simulink model "Arduino_heat_exchanger_PID"  (R2017b)
settings: Solver=VariableStepAuto  StartTime=0.0  StopTime=2400  RelTol=1e-3
values from neighbouring files (symbols this model uses):
  Area = n*A_heat_plate    (= 9.8716)    [heat_exchanger_config.m]    (also in linearization.m = 20)
  cp_H2O = 4190    [heat_exchanger_config.m]    (also in linearization.m)
  cp_wort = 4062    [heat_exchanger_config.m]    (also in linearization.m = 4000)
  HE_delay = 25    [heat_exchanger_config.m]    (also in linearization.m = 5)
  m_H2O = m_wort    (= 10)    [heat_exchanger_config.m]    (also in linearization.m = 1)
  m_wort = 10    [heat_exchanger_config.m]    (also in linearization.m = 1)
  rho_wort = 1.06    [heat_exchanger_config.m]    (also in linearization.m)
  T_H2O_in = 5    [heat_exchanger_config.m]    (also in linearization.m = 10)
  T_wort_in = 95    [heat_exchanger_config.m]    (also in linearization.m = 70)
  U = (m_dot_h_data*cp_wort*(T_wort_in-T_wort_out)*log(Delta_T2/Delta_T1))/     (Area*(Delta_T2-Delta_T1))    [heat_exchanger_config.m]    (also in linearization.m = 1000)
libraries: instrumentlib x3, simulink x1
settings Model: Creator=Alexander  LastModifiedBy=Oscar

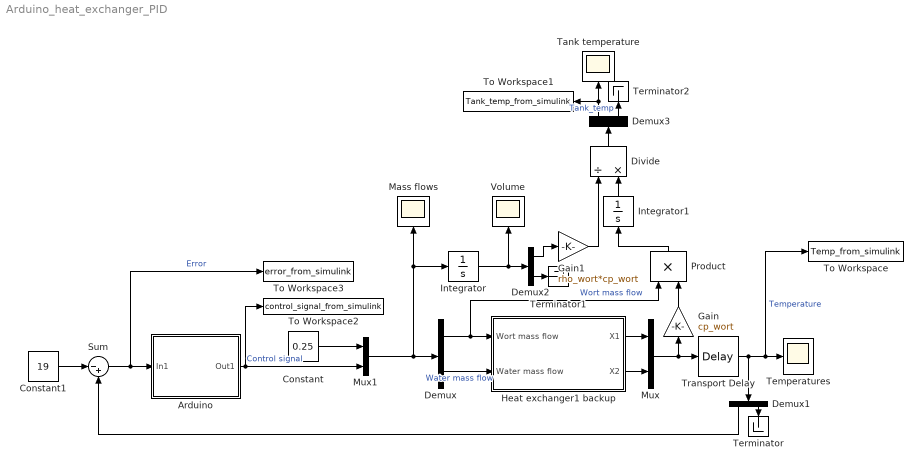
== system Arduino_heat_exchanger_PID ==
  "Arduino " : Subsystem
  Constant : Constant  Value=0.25
  Constant1 : Constant  Value=19
  Demux{,1..3} (4 alike) : Demux  Outputs=2
  Divide : Product  Inputs=/*
  Gain : Gain  Gain=cp_wort
  Gain1 : Gain  Gain=rho_wort*cp_wort
  Heat exchanger1 backup : Subsystem
  Integrator : Integrator
  Integrator1 : Integrator
  Mass flows : Scope
  Mux : Mux  Inputs=2
  Mux1 : Mux  Inputs=2
  Product : Product
  Sum : Sum  Inputs=|-+
  Tank temperature : Scope
  Temperatures : Scope
  Terminator : Terminator
  Terminator1 : Terminator
  Terminator2 : Terminator
  To Workspace : ToWorkspace  VariableName=Temp_from_simulink  SaveFormat=Timeseries  SampleTime=-1
  To Workspace1 : ToWorkspace  VariableName=Tank_temp_from_simulink  SaveFormat=Timeseries  SampleTime=-1
  To Workspace2 : ToWorkspace  VariableName=control_signal_from_simulink  SaveFormat=Timeseries  SampleTime=-1
  To Workspace3 : ToWorkspace  VariableName=error_from_simulink  SaveFormat=Timeseries  SampleTime=-1
  Transport Delay : TransportDelay  DelayTime=HE_delay
  Volume : Scope
  wires:
  Demux/2 -> Heat exchanger1 backup/2(Water mass flow)  "Water mass flow"
  Demux/1 -> Product/1, Heat exchanger1 backup/1(Wort mass flow)  "Wort mass flow"
  Mux/1 -> Gain/1, Transport Delay/1
  Integrator/1 -> Demux2/1, Volume/1
  Transport Delay/1 -> Demux1/1, To Workspace/1, Temperatures/1  "Temperature"
  Demux1/2 -> Terminator/1
  Mux1/1 -> Integrator/1, Mass flows/1, Demux/1
  Constant/1 -> Mux1/1
  Demux1/1 -> Sum/2
  Constant1/1 -> Sum/1
  Heat exchanger1 backup/1(X1) -> Mux/1
  Heat exchanger1 backup/2(X2) -> Mux/2
  Integrator1/1 -> Divide/2
  Gain1/1 -> Divide/1
  Product/1 -> Integrator1/1
  Gain/1 -> Product/2
  Demux2/1 -> Gain1/1
  Demux2/2 -> Terminator1/1
  Demux3/2 -> Terminator2/1
  Divide/1 -> Demux3/1
  Demux3/1 -> Tank temperature/1, To Workspace1/1  "Tank_temp"
  Sum/1 -> To Workspace3/1, "Arduino "/1(In1)  "Error"
  "Arduino "/1(Out1) -> Mux1/2, To Workspace2/1  "Control signal"

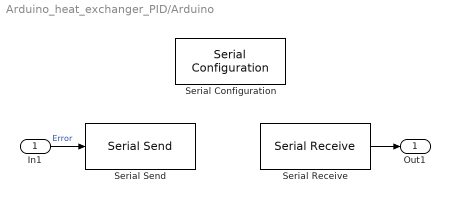
== system Arduino_heat_exchanger_PID/Arduino  ==
  In1 : Inport
  Serial Configuration : instrumentlib/Serial Configuration  Priority=-200000  ComPortMenu=<Please select a port...>  ComPort=<Please select a port...>  BaudRate=9600  DataBits=8  Parity=none  StopBits=1  FlowControl=none  Timeout=10  ByteOrder=LittleEndian
  Serial Receive : instrumentlib/Serial Receive  ComPortMenu=<Please select a port...>  ComPort=<Please select a port...>  Terminator=<none>  DataSize=[1 1]  DataType=uint8  EnableBlockingMode=on  ActionDataUnavailable=Output last received value  CustomValue=0  SampleTime=0.01
  Serial Send : instrumentlib/Serial Send  ComPortMenu=<Please select a port...>  ComPort=<Please select a port...>  Terminator=<none>  EnableBlockingMode=on
  Out1 : Outport
  wires:
  In1/1 -> Serial Send/1  "Error"
  Serial Receive/1 -> Out1/1

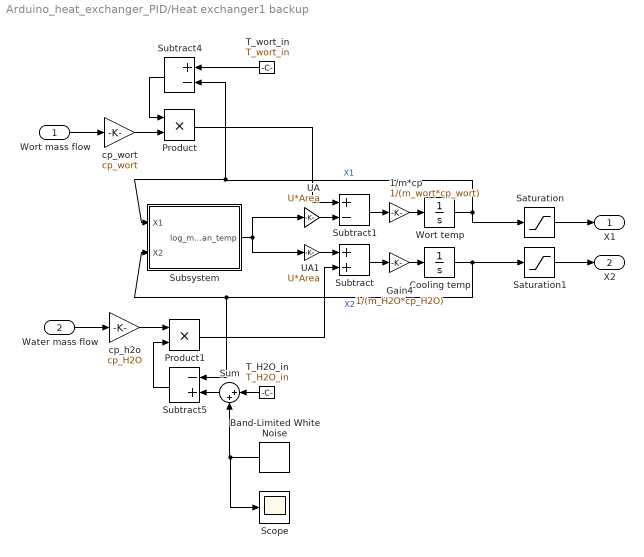
== system Arduino_heat_exchanger_PID/Heat exchanger1 backup ==
  Wort mass flow : Inport
  Water mass flow : Inport  Port=2
  "1/m*cp " : Gain  Gain=1/(m_wort*cp_wort)
  Band-Limited White Noise : simulink/Sources/Band-Limited White Noise  Cov=[5]  Ts=100  seed=[23341]
  Cooling temp : Integrator  InitialCondition=T_H2O_in-0.1
  Gain4 : Gain  Gain=1/(m_H2O*cp_H2O)
  Product : Product
  Product1 : Product
  Saturation : Saturate  UpperLimit=T_wort_in  LowerLimit=T_H2O_in
  Saturation1 : Saturate  UpperLimit=T_wort_in  LowerLimit=T_H2O_in
  Scope : Scope
  Subsystem : Subsystem
  Subtract : Sum
  Subtract1 : Sum  Inputs=+-
  Subtract4 : Sum  Inputs=+-
  Subtract5 : Sum  Inputs=-+
  Sum : Sum  Inputs=|++
  T_H2O_in : Constant  Value=T_H2O_in
  T_wort_in : Constant  Value=T_wort_in
  UA : Gain  Gain=U*Area
  "UA1 " : Gain  Gain=U*Area
  Wort temp : Integrator  InitialCondition=T_wort_in-0.1
  cp_h2o : Gain  Gain=cp_H2O
  cp_wort : Gain  Gain=cp_wort
  X1 : Outport
  X2 : Outport  Port=2
  wires:
  Cooling temp/1 -> Saturation1/1, Subtract5/1, Subsystem/2(X2)  "X2"
  "1/m*cp "/1 -> Wort temp/1
  Wort temp/1 -> Saturation/1, Subsystem/1("X1 "), Subtract4/2  "X1"
  UA/1 -> Subtract1/2
  Subtract1/1 -> "1/m*cp "/1
  Gain4/1 -> Cooling temp/1
  "UA1 "/1 -> Subtract/1
  Subtract/1 -> Gain4/1
  T_wort_in/1 -> Subtract4/1
  Subtract5/1 -> Product1/2
  Product/1 -> Subtract1/1
  Subtract4/1 -> Product/1
  Water mass flow/1 -> cp_h2o/1
  Wort mass flow/1 -> cp_wort/1
  Product1/1 -> Subtract/2
  cp_h2o/1 -> Product1/1
  cp_wort/1 -> Product/2
  Subsystem/1(log_mean_temp) -> UA/1, "UA1 "/1
  Saturation/1 -> X1/1
  Saturation1/1 -> X2/1
  Sum/1 -> Subtract5/2
  T_H2O_in/1 -> Sum/1
  Band-Limited White Noise/1 -> Scope/1, Sum/2

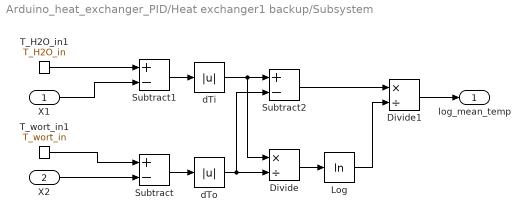
== system Arduino_heat_exchanger_PID/Heat exchanger1 backup/Subsystem ==
  "X1 " : Inport
  X2 : Inport  Port=2
  Divide : Product  Inputs=*/
  Divide1 : Product  Inputs=*/
  Log : Math  Operator=log  SaturateOnIntegerOverflow=on
  Subtract : Sum  Inputs=+-
  Subtract1 : Sum  Inputs=+-
  Subtract2 : Sum  Inputs=+-
  T_H2O_in1 : Constant  Value=T_H2O_in
  T_wort_in1 : Constant  Value=T_wort_in
  dTi : Abs
  dTo : Abs
  log_mean_temp : Outport
  wires:
  Subtract/1 -> dTo/1
  T_wort_in1/1 -> Subtract/1
  X2/1 -> Subtract/2
  Subtract1/1 -> dTi/1
  "X1 "/1 -> Subtract1/2
  T_H2O_in1/1 -> Subtract1/1
  dTo/1 -> Subtract2/2, Divide/2
  dTi/1 -> Subtract2/1, Divide/1
  Divide/1 -> Log/1
  Log/1 -> Divide1/2
  Divide1/1 -> log_mean_temp/1
  Subtract2/1 -> Divide1/1
